simulink model "sampleModel1934"  (R2023a)
settings: Solver=VariableStepAuto  StartTime=0.0  StopTime=10.0  RelTol=1e-3
libraries: hdlsllib x7, simulink x2
settings Model: Creator=user1  LastModifiedBy=user1

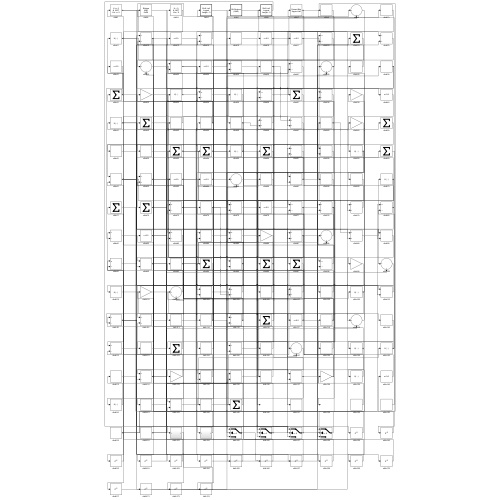
[thumbnail: Simulink's stored preview of the top-level diagram]
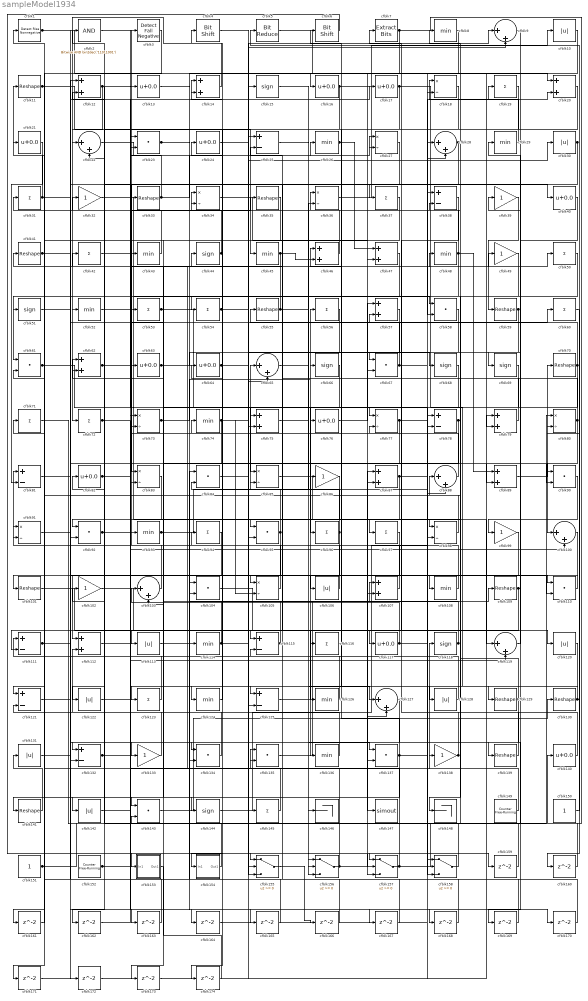
== system sampleModel1934 ==
  cfblk1 : hdlsllib/Logic and Bit Operations/Detect Rise Nonnegative  vinit=0  OutDataTypeStr=boolean
  cfblk{10,30,106,113,120,122,128,131,142} (9 alike) : Abs  SaturateOnIntegerOverflow=off
  cfblk{9,22,28,65,88,100,103,119,127} (9 alike) : Sum  Inputs=|++
  cfblk{11,33,35,41,55,59,70,101,109,129..130,139,141} (13 alike) : Reshape
  cfblk{32,39,49,86,99,102,133,138} (8 alike) : Gain
  cfblk{23,58,61,67,84,90,92,95,104,110,134..135,137,143} (14 alike) : DotProduct  OutDataTypeStr=Inherit: Inherit via internal rule
  cfblk{18,27,34,36,73,77,80,83,85,91,98,105} (12 alike) : Product  Inputs=*/  RndMeth=Zero  SaturateOnIntegerOverflow=on
  cfblk{12,14,20,46..47,57,62,75,79,87,89,107,112} (13 alike) : Sum
  cfblk{8,26,29,43,45,48,52,74,93,108,114,124,126,136} (14 alike) : MinMax
  cfblk{25,38,78,81,111,115,121,125,132} (9 alike) : Sum  Inputs=+-
  cfblk{19,31,37,42,50,53..54,56,60,71..72,94,96..97,116,123,145} (17 alike) : Sum  Inputs=+
  cfblk{13,16..17,21,24,40,63..64,76,82,117,140} (12 alike) : Bias  Bias=0.0  SaturateOnIntegerOverflow=off
  cfblk{15,44,51,66,68..69,118,144} (8 alike) : Signum
  cfblk146 : Terminator
  cfblk147 : ToWorkspace  VariableName=simout  SaveFormat=Timeseries  SampleTime=-1
  cfblk148 : Terminator
  cfblk149 : hdlsllib/Sources/Counter Free-Running  NumBits=16  tsamp=-1
  cfblk150 : Constant  SampleTime=-1
  cfblk151 : Constant  SampleTime=-1
  cfblk152 : hdlsllib/Sources/Counter Free-Running  NumBits=16  tsamp=-1
  cfblk153 : Subsystem
      settings: LibrarySourceBlock=|
      | hdlsllib/Ports &
      | Subsystems/Subsystem
  cfblk154 : Subsystem
      settings: LibrarySourceBlock=|
      | hdlsllib/Ports &
      | Subsystems/Subsystem
  cfblk{155..158} (4 alike) : Switch  SaturateOnIntegerOverflow=off  InputSameDT=off
  cfblk{159..174} (16 alike) : Delay  SampleTime=1
  cfblk2 : simulink/Logic and Bit Operations/Bitwise Operator  logicop=AND  UseBitMask=on  BitMask=bin2dec('11011001')  BitMaskRealWorld=Stored Integer
      settings: LibrarySourceBlock=|
      | hdlsllib/Logic and Bit
      | Operations/Bitwise
      | Operator
  cfblk3 : hdlsllib/Logic and Bit Operations/Detect Fall Negative  vinit=0  OutDataTypeStr=boolean
  cfblk4 : hdlsllib/Logic and Bit Operations/Bit Shift  mode=Shift Left Logical  N=0
  cfblk5 : hdlsllib/Logic and Bit Operations/Bit Reduce  mode=AND
  cfblk6 : hdlsllib/Logic and Bit Operations/Bit Shift  mode=Shift Left Logical  N=0
  cfblk7 : simulink/Logic and Bit Operations/Extract Bits  bitsToExtract=Upper half  numBits=8  bitIdxRange=[0 7]  outScalingMode=Preserve fixed-point scaling
      settings: LibrarySourceBlock=|
      | hdlsllib/Logic and Bit
      | Operations/Extract Bits
  wires:
  cfblk88/1 -> cfblk74/1
  cfblk78/1 -> cfblk97/1, cfblk103/2
  cfblk103/1 -> cfblk3/1
  cfblk17/1 -> cfblk125/1, cfblk76/1
  cfblk145/1 -> cfblk48/1
  cfblk14/1 -> cfblk72/1
  cfblk149/1 -> cfblk118/1
  cfblk72/1 -> cfblk27/2, cfblk165/1
  cfblk100/1 -> cfblk112/1
  cfblk96/1 -> cfblk65/1, cfblk106/1
  cfblk118/1 -> cfblk62/1, cfblk77/2
  cfblk48/1 -> cfblk115/1, cfblk89/1, cfblk21/1
  cfblk137/1 -> cfblk78/1, cfblk141/1, cfblk46/1
  cfblk26/1 -> cfblk47/1, cfblk116/1
  cfblk28/1 -> cfblk16/1, cfblk156/3
  cfblk53/1 -> cfblk68/1, cfblk86/1
  cfblk12/1 -> cfblk22/1, cfblk122/1, cfblk75/2
  cfblk83/1 -> cfblk142/1
  cfblk66/1 -> cfblk85/1
  cfblk150/1 -> cfblk5/1
  cfblk125/1 -> cfblk56/1
  cfblk7/1 -> cfblk140/1, cfblk47/2
  cfblk105/1 -> cfblk24/1
  cfblk71/1 -> cfblk139/1
  cfblk115/1 -> cfblk93/1, cfblk44/1
  cfblk68/1 -> cfblk113/1
  cfblk127/1 -> cfblk133/1
  cfblk23/1 -> cfblk104/1, cfblk110/2
  cfblk120/1 -> cfblk129/1
  cfblk77/1 -> cfblk19/1, cfblk155/3
  cfblk27/1 -> cfblk92/1
  cfblk51/1 -> cfblk92/2
  cfblk87/1 -> cfblk88/2, cfblk134/1, cfblk162/1
  cfblk64/1 -> cfblk15/1, cfblk14/1
  cfblk128/1 -> cfblk4/1
  cfblk132/1 -> cfblk42/1, cfblk135/2, cfblk14/2
  cfblk11/1 -> cfblk45/1, cfblk107/2
  cfblk16/1 -> cfblk20/1, cfblk54/1
  cfblk70/1 -> cfblk96/1, cfblk25/2, cfblk137/2
  cfblk144/1 -> cfblk28/1
  cfblk29/1 -> cfblk18/1
  cfblk135/1 -> cfblk109/1
  cfblk107/1 -> cfblk81/1
  cfblk37/1 -> cfblk143/1
  cfblk32/1 -> cfblk119/1
  cfblk97/1 -> cfblk132/1
  cfblk85/1 -> cfblk98/1
  cfblk15/1 -> cfblk127/1
  cfblk59/1 -> cfblk125/2, cfblk67/2
  cfblk39/1 -> cfblk59/1
  cfblk52/1 -> cfblk95/1
  cfblk119/1 -> cfblk39/1
  cfblk33/1 -> cfblk23/1, cfblk27/1
  cfblk117/1 -> cfblk50/1, cfblk103/1
  cfblk123/1 -> cfblk111/1
  cfblk75/1 -> cfblk156/1
  cfblk2/1 -> cfblk40/1
  cfblk42/1 -> cfblk58/1
  cfblk45/1 -> cfblk61/1, cfblk46/2
  cfblk156/1 -> cfblk87/1, cfblk91/2
  cfblk91/1 -> cfblk60/1
  cfblk38/1 -> cfblk117/1
  cfblk61/1 -> cfblk114/1, cfblk17/1, cfblk90/1, cfblk90/2
  cfblk139/1 -> cfblk38/2
  cfblk69/1 -> cfblk128/1
  cfblk98/1 -> cfblk71/1
  cfblk34/1 -> cfblk127/2
  cfblk108/1 -> cfblk55/1
  cfblk124/1 -> cfblk84/2
  cfblk89/1 -> cfblk70/1
  cfblk62/1 -> cfblk146/1, cfblk158/1
  cfblk134/1 -> cfblk91/1
  cfblk143/1 -> cfblk130/1
  cfblk31/1 -> cfblk11/1, cfblk89/2
  cfblk109/1 -> cfblk29/1, cfblk111/2
  cfblk126/1 -> cfblk12/2
  cfblk49/1 -> cfblk148/1
  cfblk58/1 -> cfblk95/2
  cfblk8/1 -> cfblk104/2
  cfblk1/1 -> cfblk79/2, cfblk37/1
  cfblk30/1 -> cfblk83/1, cfblk105/1
  cfblk102/1 -> cfblk136/1
  cfblk116/1 -> cfblk36/1
  cfblk158/1 -> cfblk143/2
  cfblk93/1 -> cfblk20/2, cfblk36/2
  cfblk21/1 -> cfblk81/2
  cfblk94/1 -> cfblk101/1
  cfblk73/1 -> cfblk66/1, cfblk157/2
  cfblk67/1 -> cfblk28/2, cfblk6/1
  cfblk6/1 -> cfblk153/1(In1)
  cfblk101/1 -> cfblk145/1
  cfblk130/1 -> cfblk123/1, cfblk80/2
  cfblk110/1 -> cfblk108/1
  cfblk129/1 -> cfblk8/1, cfblk132/2
  cfblk136/1 -> cfblk112/2
  cfblk63/1 -> cfblk77/1, cfblk67/1
  cfblk157/1 -> cfblk102/1, cfblk80/1
  cfblk5/1 -> cfblk58/2
  cfblk154/1(Out1) -> cfblk82/1
  cfblk10/1 -> cfblk18/2
  cfblk82/1 -> cfblk35/1, cfblk100/2
  cfblk95/1 -> cfblk154/1(In1), cfblk64/1
  cfblk20/1 -> cfblk52/1
  cfblk22/1 -> cfblk26/1
  cfblk80/1 -> cfblk41/1, cfblk100/1
  cfblk35/1 -> cfblk121/1
  cfblk55/1 -> cfblk87/2, cfblk51/1
  cfblk76/1 -> cfblk57/1
  cfblk114/1 -> cfblk43/1, cfblk62/2, cfblk158/3
  cfblk122/1 -> cfblk119/2
  cfblk47/1 -> cfblk124/1
  cfblk19/1 -> cfblk144/1
  cfblk40/1 -> cfblk69/1
  cfblk9/1 -> cfblk99/1
  cfblk84/1 -> cfblk30/1
  cfblk4/1 -> cfblk157/1
  cfblk18/1 -> cfblk23/2
  cfblk141/1 -> cfblk131/1
  cfblk54/1 -> cfblk120/1, cfblk9/2
  cfblk142/1 -> cfblk138/1
  cfblk113/1 -> cfblk107/1
  cfblk50/1 -> cfblk126/1
  cfblk104/1 -> cfblk147/1
  cfblk152/1 -> cfblk135/1, cfblk49/1
  cfblk56/1 -> cfblk75/1
  cfblk36/1 -> cfblk10/1
  cfblk106/1 -> cfblk32/1
  cfblk44/1 -> cfblk31/1, cfblk34/1
  cfblk74/1 -> cfblk25/1, cfblk134/2, cfblk105/2
  cfblk138/1 -> cfblk57/2, cfblk94/1
  cfblk111/1 -> cfblk155/1, cfblk13/1, cfblk157/3
  cfblk133/1 -> cfblk121/2
  cfblk151/1 -> cfblk78/2, cfblk63/1
  cfblk65/1 -> cfblk137/1
  cfblk140/1 -> cfblk73/2
  cfblk24/1 -> cfblk9/1
  cfblk57/1 -> cfblk156/2
  cfblk79/1 -> cfblk7/1
  cfblk43/1 -> cfblk33/1
  cfblk46/1 -> cfblk2/1
  cfblk41/1 -> cfblk110/1, cfblk168/1
  cfblk92/1 -> cfblk155/2, cfblk34/2
  cfblk25/1 -> cfblk159/1
  cfblk159/1 -> cfblk88/1
  cfblk60/1 -> cfblk160/1
  cfblk160/1 -> cfblk22/2
  cfblk99/1 -> cfblk161/1
  cfblk161/1 -> cfblk1/1
  cfblk162/1 -> cfblk83/2
  cfblk121/1 -> cfblk163/1
  cfblk163/1 -> cfblk12/1
  cfblk112/1 -> cfblk164/1
  cfblk164/1 -> cfblk98/2
  cfblk165/1 -> cfblk84/1
  cfblk155/1 -> cfblk166/1
  cfblk166/1 -> cfblk85/2
  cfblk13/1 -> cfblk167/1
  cfblk167/1 -> cfblk115/2
  cfblk168/1 -> cfblk158/2
  cfblk90/1 -> cfblk169/1
  cfblk169/1 -> cfblk61/2
  cfblk81/1 -> cfblk170/1
  cfblk170/1 -> cfblk73/1
  cfblk3/1 -> cfblk171/1
  cfblk171/1 -> cfblk79/1
  cfblk131/1 -> cfblk172/1
  cfblk172/1 -> cfblk65/2
  cfblk153/1(Out1) -> cfblk173/1
  cfblk173/1 -> cfblk38/1
  cfblk86/1 -> cfblk174/1
  cfblk174/1 -> cfblk53/1

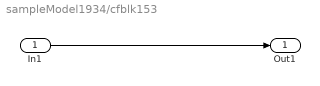
== system sampleModel1934/cfblk153 ==
  In1 : Inport
  Out1 : Outport
  wires:
  In1/1 -> Out1/1

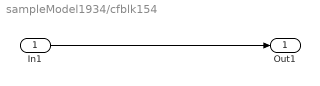
== system sampleModel1934/cfblk154 ==
  In1 : Inport
  Out1 : Outport
  wires:
  In1/1 -> Out1/1
